simulink model "bh_compare_hand_to_SM_quad_pend"  (R2020b)
settings: Solver=ode23t  StartTime=0.0  StopTime=50  FixedStep=0.001  RelTol=1e-5  EnableMultiTasking=on
undefined symbols (not defined in the file): K, P_elec, P_mot, P_one_prop, P_pend, P_rot, P_veh, P_veh_no_props, sigbuilder_block, X, xme_dot_0, Y, Z
libraries: fl_lib x85, simulink_extras x42, nesl_utility x39, sm_lib x29, pid_lib x8, fl_ps_legacy_lib x7, simulink x6
(part 2 of 5)

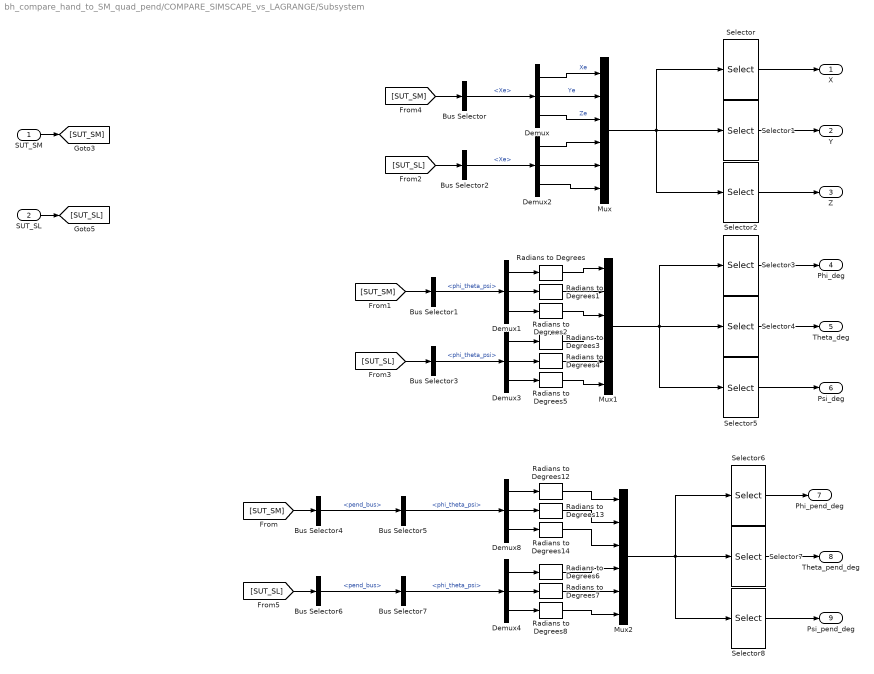
== system bh_compare_hand_to_SM_quad_pend/COMPARE_SIMSCAPE_vs_LAGRANGE/Subsystem ==
  SUT_SM : Inport
  SUT_SL : Inport  Port=2
  Bus Selector : BusSelector  OutputSignals=Xe
  Bus Selector{1,3,5,7} (4 alike) : BusSelector  OutputSignals=phi_theta_psi
  Bus Selector2 : BusSelector  OutputSignals=Xe
  Bus Selector4 : BusSelector  OutputSignals=pend_bus
  Bus Selector6 : BusSelector  OutputSignals=pend_bus
  Demux{,1..4,8} (6 alike) : Demux  Outputs=3
  Mux : Mux  Inputs=6
  Mux1 : Mux  Inputs=6
  Mux2 : Mux  Inputs=6
  Radians to Degrees{,1..8,12..14} (12 alike) : simulink_extras/Transformations/Radians to Degrees
  Selector : Selector  InputPortWidth=6  IndexOptions=Index vector (dialog)  Indices=[1 4]  OutputSizes=1
  Selector1 : Selector  InputPortWidth=6  IndexOptions=Index vector (dialog)  Indices=[2 5]  OutputSizes=1
  Selector2 : Selector  InputPortWidth=6  IndexOptions=Index vector (dialog)  Indices=[3 6]  OutputSizes=1
  Selector3 : Selector  InputPortWidth=6  IndexOptions=Index vector (dialog)  Indices=[1 4]  OutputSizes=1
  Selector4 : Selector  InputPortWidth=6  IndexOptions=Index vector (dialog)  Indices=[2 5]  OutputSizes=1
  Selector5 : Selector  InputPortWidth=6  IndexOptions=Index vector (dialog)  Indices=[3 6]  OutputSizes=1
  Selector6 : Selector  InputPortWidth=6  IndexOptions=Index vector (dialog)  Indices=[1 4]  OutputSizes=1
  Selector7 : Selector  InputPortWidth=6  IndexOptions=Index vector (dialog)  Indices=[2 5]  OutputSizes=1
  Selector8 : Selector  InputPortWidth=6  IndexOptions=Index vector (dialog)  Indices=[3 6]  OutputSizes=1
  X : Outport  VectorParamsAs1DForOutWhenUnconnected=off
  Y : Outport  Port=2  VectorParamsAs1DForOutWhenUnconnected=off
  Z : Outport  Port=3  VectorParamsAs1DForOutWhenUnconnected=off
  Phi_deg : Outport  Port=4  VectorParamsAs1DForOutWhenUnconnected=off
  Theta_deg : Outport  Port=5  VectorParamsAs1DForOutWhenUnconnected=off
  Psi_deg : Outport  Port=6  VectorParamsAs1DForOutWhenUnconnected=off
  Phi_pend_deg : Outport  Port=7  VectorParamsAs1DForOutWhenUnconnected=off
  Theta_pend_deg : Outport  Port=8  VectorParamsAs1DForOutWhenUnconnected=off
  Psi_pend_deg : Outport  Port=9  VectorParamsAs1DForOutWhenUnconnected=off
  wires:
  SUT_SL/1 -> [SUT_SL]
  SUT_SM/1 -> [SUT_SM]
  Demux8/2 -> Radians to Degrees13/1
  [SUT_SM] -> Bus Selector1/1
  Bus Selector1/1 -> Demux1/1  "<phi_theta_psi>"
  Bus Selector/1 -> Demux/1  "<Xe>"
  Demux1/2 -> Radians to Degrees1/1
  Demux8/3 -> Radians to Degrees14/1
  [SUT_SM] -> Bus Selector4/1
  Demux8/1 -> Radians to Degrees12/1
  [SUT_SM] -> Bus Selector/1
  Demux1/1 -> Radians to Degrees/1
  Demux1/3 -> Radians to Degrees2/1
  [SUT_SL] -> Bus Selector2/1
  Bus Selector2/1 -> Demux2/1  "<Xe>"
  Demux3/1 -> Radians to Degrees3/1
  [SUT_SL] -> Bus Selector3/1
  Bus Selector3/1 -> Demux3/1  "<phi_theta_psi>"
  Demux3/2 -> Radians to Degrees4/1
  Demux3/3 -> Radians to Degrees5/1
  Bus Selector4/1 -> Bus Selector5/1  "<pend_bus>"
  Bus Selector5/1 -> Demux8/1  "<phi_theta_psi>"
  [SUT_SL] -> Bus Selector6/1
  Demux4/2 -> Radians to Degrees7/1
  Demux4/1 -> Radians to Degrees6/1
  Demux4/3 -> Radians to Degrees8/1
  Bus Selector6/1 -> Bus Selector7/1  "<pend_bus>"
  Bus Selector7/1 -> Demux4/1  "<phi_theta_psi>"
  Demux2/2 -> Mux/5
  Demux2/3 -> Mux/6
  Demux2/1 -> Mux/4
  Demux/3 -> Mux/3  "Ze"
  Demux/2 -> Mux/2  "Ye"
  Demux/1 -> Mux/1  "Xe"
  Radians to Degrees5/1 -> Mux1/6
  Radians to Degrees4/1 -> Mux1/5
  Radians to Degrees3/1 -> Mux1/4
  Radians to Degrees2/1 -> Mux1/3
  Radians to Degrees1/1 -> Mux1/2
  Radians to Degrees/1 -> Mux1/1
  Radians to Degrees12/1 -> Mux2/1
  Radians to Degrees13/1 -> Mux2/2
  Radians to Degrees14/1 -> Mux2/3
  Radians to Degrees6/1 -> Mux2/4
  Radians to Degrees7/1 -> Mux2/5
  Radians to Degrees8/1 -> Mux2/6
  Mux2/1 -> Selector8/1, Selector6/1, Selector7/1
  Mux/1 -> Selector/1, Selector2/1, Selector1/1
  Mux1/1 -> Selector5/1, Selector3/1, Selector4/1
  Selector2/1 -> Z/1
  Selector1/1 -> Y/1
  Selector/1 -> X/1
  Selector5/1 -> Psi_deg/1
  Selector4/1 -> Theta_deg/1
  Selector3/1 -> Phi_deg/1
  Selector6/1 -> Phi_pend_deg/1
  Selector8/1 -> Psi_pend_deg/1
  Selector7/1 -> Theta_pend_deg/1

== system bh_compare_hand_to_SM_quad_pend/CONT_SYS W_MOT_CMDS1/MOTOR_sys ==
  w_CMD : Inport
  Demux : Demux
  MOTOR_1 : Subsystem
      mask Display: image('bh_PIC_MOTOR.jpg');
  MOTOR_2 : Subsystem
      mask Display: image('bh_PIC_MOTOR.jpg');
  MOTOR_3 : Subsystem
      mask Display: image('bh_PIC_MOTOR.jpg');
  MOTOR_4 : Subsystem
      mask Display: image('bh_PIC_MOTOR.jpg');
  Mux : Mux
  w CMD vs Actual : Scope  NumInputPorts=4
  w_MUX : Subsystem
  w : Outport  VectorParamsAs1DForOutWhenUnconnected=off
  wires:
  MOTOR_4/1(w) -> Mux/4
  MOTOR_3/1(w) -> Mux/3
  MOTOR_2/1(w) -> Mux/2
  MOTOR_1/1(w) -> Mux/1
  Demux/1 -> MOTOR_1/1(w_CMD)
  Demux/2 -> MOTOR_2/1(w_CMD)
  Demux/3 -> MOTOR_3/1(w_CMD)
  Demux/4 -> MOTOR_4/1(w_CMD)
  w_CMD/1 -> [W_CMD], Demux/1
  w_MUX/4(w4) -> w CMD vs Actual/4
  w_MUX/2(w2) -> w CMD vs Actual/2
  w_MUX/3(w3) -> w CMD vs Actual/3
  w_MUX/1(w1) -> w CMD vs Actual/1
  [W_CMD] -> w_MUX/1(W_CMD)
  Mux/1 -> w_MUX/2(W), w/1

== system bh_compare_hand_to_SM_quad_pend/CONT_SYS W_MOT_CMDS1/SIGN_CONVENTIONS ==

== system bh_compare_hand_to_SM_quad_pend/CONT_SYS W_MOT_CMDS1/W2_checker ==
  w2_CMD : Inport
  Assertion{,1..3} (4 alike) : Assertion
  Compare To Constant : simulink/Logic and Bit Operations/Compare To Constant  relop=>=  const=0  OutDataTypeStr=boolean
  Demux : Demux
  w2 : Outport  VectorParamsAs1DForOutWhenUnconnected=off
  wires:
  w2_CMD/1 -> w2/1, Compare To Constant/1
  Compare To Constant/1 -> Demux/1
  Demux/1 -> Assertion/1
  Demux/4 -> Assertion3/1
  Demux/3 -> Assertion2/1
  Demux/2 -> Assertion1/1

== system bh_compare_hand_to_SM_quad_pend/CONT_SYS W_MOT_CMDS1/w_to_RPS1 ==
  w : Inport
  Constant : Constant  Value=3.141592653589793
  Gain1 : Gain  Gain=2
  Product : Product  Inputs=*/
  RPS : Outport
  wires:
  Product/1 -> RPS/1
  Gain1/1 -> Product/2  "2PI"
  Constant/1 -> Gain1/1
  w/1 -> Product/1  "w_per_sec"

== system bh_compare_hand_to_SM_quad_pend/CONT_SYS W_MOT_CMDS2/PRE_FILTERS ==
  w_in : Inport
  Demux : Demux
  Mux : Mux
  Reshape2 : Reshape  OutputDimensionality=Column vector (2-D)
  Terminator{,1..3} (4 alike) : Terminator
  prefilter : Subsystem  mask(Derivative Estimation){wn=2*pi*5, p=1}
      mask prompts: wn "Natural frequency, wn (rad/sec)"; p "Damping ratio, p"
      mask help:
      | A simple derivative estimator using a 2nd order representation between input and output.
      |
      | The integrators use a discrete FORWARd Euler rule, and a sample time needs to be specified.
      mask init:
      | str1 = sprintf('wn = %.2f', wn);
      | str2 = sprintf('p  = %.2f', p);
      | %str3 = sprintf('dt = %.2f', dt);
      | %str = char(str1,str2,str3);
      | %str3 = sprintf('dt = %.2f', dt);
      | str = char(str1,str2);
      mask Display: disp(str)
  prefilter1 : Subsystem  mask(Derivative Estimation){wn=2*pi*5, p=1}
      mask prompts: wn "Natural frequency, wn (rad/sec)"; p "Damping ratio, p"
      mask help:
      | A simple derivative estimator using a 2nd order representation between input and output.
      |
      | The integrators use a discrete FORWARd Euler rule, and a sample time needs to be specified.
      mask init:
      | str1 = sprintf('wn = %.2f', wn);
      | str2 = sprintf('p  = %.2f', p);
      | %str3 = sprintf('dt = %.2f', dt);
      | %str = char(str1,str2,str3);
      | %str3 = sprintf('dt = %.2f', dt);
      | str = char(str1,str2);
      mask Display: disp(str)
  prefilter2 : Subsystem  mask(Derivative Estimation){wn=2*pi*5, p=1}
      mask prompts: wn "Natural frequency, wn (rad/sec)"; p "Damping ratio, p"
      mask help:
      | A simple derivative estimator using a 2nd order representation between input and output.
      |
      | The integrators use a discrete FORWARd Euler rule, and a sample time needs to be specified.
      mask init:
      | str1 = sprintf('wn = %.2f', wn);
      | str2 = sprintf('p  = %.2f', p);
      | %str3 = sprintf('dt = %.2f', dt);
      | %str = char(str1,str2,str3);
      | %str3 = sprintf('dt = %.2f', dt);
      | str = char(str1,str2);
      mask Display: disp(str)
  prefilter3 : Subsystem  mask(Derivative Estimation){wn=2*pi*5, p=1}
      mask prompts: wn "Natural frequency, wn (rad/sec)"; p "Damping ratio, p"
      mask help:
      | A simple derivative estimator using a 2nd order representation between input and output.
      |
      | The integrators use a discrete FORWARd Euler rule, and a sample time needs to be specified.
      mask init:
      | str1 = sprintf('wn = %.2f', wn);
      | str2 = sprintf('p  = %.2f', p);
      | %str3 = sprintf('dt = %.2f', dt);
      | %str = char(str1,str2,str3);
      | %str3 = sprintf('dt = %.2f', dt);
      | str = char(str1,str2);
      mask Display: disp(str)
  w CMD vs Actual : Scope  NumInputPorts=4
  w_MUX : Subsystem
  w : Outport  VectorParamsAs1DForOutWhenUnconnected=off
  wires:
  prefilter1/2(U_DOT) -> Terminator1/1
  prefilter/2(U_DOT) -> Terminator/1
  prefilter2/2(U_DOT) -> Terminator2/1
  prefilter3/2(U_DOT) -> Terminator3/1
  w_in/1 -> [W_CMD], Demux/1
  Demux/1 -> prefilter/1(U)
  Demux/2 -> prefilter1/1(U)
  Demux/3 -> prefilter2/1(U)
  Demux/4 -> prefilter3/1(U)
  prefilter/1(U_filt) -> Mux/1
  prefilter1/1(U_filt) -> Mux/2
  prefilter2/1(U_filt) -> Mux/3
  prefilter3/1(U_filt) -> Mux/4
  Mux/1 -> Reshape2/1
  Reshape2/1 -> w_MUX/2(W), w/1
  w_MUX/3(w3) -> w CMD vs Actual/3
  w_MUX/2(w2) -> w CMD vs Actual/2
  w_MUX/4(w4) -> w CMD vs Actual/4
  [W_CMD] -> w_MUX/1(W_CMD)
  w_MUX/1(w1) -> w CMD vs Actual/1

== system bh_compare_hand_to_SM_quad_pend/CONT_SYS W_MOT_CMDS2/SIGN_CONVENTIONS ==

== system bh_compare_hand_to_SM_quad_pend/CONT_SYS W_MOT_CMDS2/W2_checker ==
  w2_CMD : Inport
  Assertion{,1..3} (4 alike) : Assertion
  Compare To Constant : simulink/Logic and Bit Operations/Compare To Constant  relop=>=  const=0  OutDataTypeStr=boolean
  Demux : Demux
  w2 : Outport  VectorParamsAs1DForOutWhenUnconnected=off
  wires:
  w2_CMD/1 -> w2/1, Compare To Constant/1
  Compare To Constant/1 -> Demux/1
  Demux/1 -> Assertion/1
  Demux/4 -> Assertion3/1
  Demux/3 -> Assertion2/1
  Demux/2 -> Assertion1/1

== system bh_compare_hand_to_SM_quad_pend/CONT_SYS W_MOT_CMDS2/w_to_RPS1 ==
  w : Inport
  Constant : Constant  Value=3.141592653589793
  Gain1 : Gain  Gain=2
  Product : Product  Inputs=*/
  RPS : Outport
  wires:
  Product/1 -> RPS/1
  Gain1/1 -> Product/2  "2PI"
  Constant/1 -> Gain1/1
  w/1 -> Product/1  "w_per_sec"

== system bh_compare_hand_to_SM_quad_pend/EYES_PROP_and_VEH/THRUST_FUSE ==
  REF : Inport
  p1_b : Inport  Port=2
  p2_b : Inport  Port=3
  p3_b : Inport  Port=4
  p4_b : Inport  Port=5
  Bus Selector{,1..3} (4 alike) : BusSelector  OutputSignals=Thrust_on_veh
  Mux{,1..3} (4 alike) : Mux  Inputs=2
  Selector : Selector  InputPortWidth=4  IndexOptions=Index vector (dialog)  Indices=1  OutputSizes=1
  Selector1 : Selector  InputPortWidth=4  IndexOptions=Index vector (dialog)  Indices=2  OutputSizes=1
  Selector2 : Selector  InputPortWidth=4  IndexOptions=Index vector (dialog)  Indices=3  OutputSizes=1
  Selector3 : Selector  InputPortWidth=4  IndexOptions=Index vector (dialog)  Indices=4  OutputSizes=1
  Out1 : Outport  VectorParamsAs1DForOutWhenUnconnected=off
  Out2 : Outport  Port=2  VectorParamsAs1DForOutWhenUnconnected=off
  Out3 : Outport  Port=3  VectorParamsAs1DForOutWhenUnconnected=off
  Out4 : Outport  Port=4  VectorParamsAs1DForOutWhenUnconnected=off
  wires:
  Mux/1 -> Out4/1
  Mux1/1 -> Out3/1
  Mux2/1 -> Out2/1
  Mux3/1 -> Out1/1
  p1_b/1 -> Bus Selector/1
  Bus Selector/1 -> Mux3/2  "<Thrust_on_veh>"
  Selector/1 -> Mux3/1
  Selector1/1 -> Mux2/1
  Selector2/1 -> Mux1/1
  Selector3/1 -> Mux/1
  REF/1 -> Selector3/1, Selector2/1, Selector1/1, Selector/1
  p2_b/1 -> Bus Selector1/1
  Bus Selector1/1 -> Mux2/2  "<Thrust_on_veh>"
  p3_b/1 -> Bus Selector2/1
  Bus Selector2/1 -> Mux1/2  "<Thrust_on_veh>"
  p4_b/1 -> Bus Selector3/1
  Bus Selector3/1 -> Mux/2  "<Thrust_on_veh>"

== system bh_compare_hand_to_SM_quad_pend/EYES_PROP_and_VEH/TQ_FUSE ==
  REF : Inport
  p1_b : Inport  Port=2
  p2_b : Inport  Port=3
  p3_b : Inport  Port=4
  p4_b : Inport  Port=5
  Bus Selector{,1..3} (4 alike) : BusSelector  OutputSignals=Torque_on_veh
  Mux{,1..3} (4 alike) : Mux  Inputs=2
  Selector : Selector  InputPortWidth=4  IndexOptions=Index vector (dialog)  Indices=1  OutputSizes=1
  Selector1 : Selector  InputPortWidth=4  IndexOptions=Index vector (dialog)  Indices=2  OutputSizes=1
  Selector2 : Selector  InputPortWidth=4  IndexOptions=Index vector (dialog)  Indices=3  OutputSizes=1
  Selector3 : Selector  InputPortWidth=4  IndexOptions=Index vector (dialog)  Indices=4  OutputSizes=1
  Out1 : Outport  VectorParamsAs1DForOutWhenUnconnected=off
  Out2 : Outport  Port=2  VectorParamsAs1DForOutWhenUnconnected=off
  Out3 : Outport  Port=3  VectorParamsAs1DForOutWhenUnconnected=off
  Out4 : Outport  Port=4  VectorParamsAs1DForOutWhenUnconnected=off
  wires:
  Mux/1 -> Out4/1
  Mux1/1 -> Out3/1
  Mux2/1 -> Out2/1
  Mux3/1 -> Out1/1
  p1_b/1 -> Bus Selector/1
  Bus Selector/1 -> Mux3/2  "<Torque_on_veh>"
  Selector/1 -> Mux3/1
  Selector1/1 -> Mux2/1
  Selector2/1 -> Mux1/1
  Selector3/1 -> Mux/1
  REF/1 -> Selector3/1, Selector2/1, Selector1/1, Selector/1
  p2_b/1 -> Bus Selector1/1
  Bus Selector1/1 -> Mux2/2  "<Torque_on_veh>"
  p3_b/1 -> Bus Selector2/1
  Bus Selector2/1 -> Mux1/2  "<Torque_on_veh>"
  p4_b/1 -> Bus Selector3/1
  Bus Selector3/1 -> Mux/2  "<Torque_on_veh>"

== system bh_compare_hand_to_SM_quad_pend/EYES_PROP_and_VEH/w_FUSE ==
  REF : Inport
  p1_b : Inport  Port=2
  p2_b : Inport  Port=3
  p3_b : Inport  Port=4
  p4_b : Inport  Port=5
  Bus Selector{,1..3} (4 alike) : BusSelector  OutputSignals=w_prop
  Mux{,1..3} (4 alike) : Mux  Inputs=2
  Selector : Selector  InputPortWidth=4  IndexOptions=Index vector (dialog)  Indices=1  OutputSizes=1
  Selector1 : Selector  InputPortWidth=4  IndexOptions=Index vector (dialog)  Indices=2  OutputSizes=1
  Selector2 : Selector  InputPortWidth=4  IndexOptions=Index vector (dialog)  Indices=3  OutputSizes=1
  Selector3 : Selector  InputPortWidth=4  IndexOptions=Index vector (dialog)  Indices=4  OutputSizes=1
  Out1 : Outport  VectorParamsAs1DForOutWhenUnconnected=off
  Out2 : Outport  Port=2  VectorParamsAs1DForOutWhenUnconnected=off
  Out3 : Outport  Port=3  VectorParamsAs1DForOutWhenUnconnected=off
  Out4 : Outport  Port=4  VectorParamsAs1DForOutWhenUnconnected=off
  wires:
  Mux/1 -> Out4/1
  Mux1/1 -> Out3/1
  Mux2/1 -> Out2/1
  Mux3/1 -> Out1/1
  p1_b/1 -> Bus Selector/1
  Bus Selector/1 -> Mux3/2  "<w_prop>"
  Selector/1 -> Mux3/1
  Selector1/1 -> Mux2/1
  Selector2/1 -> Mux1/1
  Selector3/1 -> Mux/1
  REF/1 -> Selector3/1, Selector2/1, Selector1/1, Selector/1
  Bus Selector1/1 -> Mux2/2  "<w_prop>"
  p2_b/1 -> Bus Selector1/1
  Bus Selector2/1 -> Mux1/2  "<w_prop>"
  p3_b/1 -> Bus Selector2/1
  Bus Selector3/1 -> Mux/2  "<w_prop>"
  p4_b/1 -> Bus Selector3/1

== system bh_compare_hand_to_SM_quad_pend/MODEL_SYS/SIGN_CONVENTIONS ==

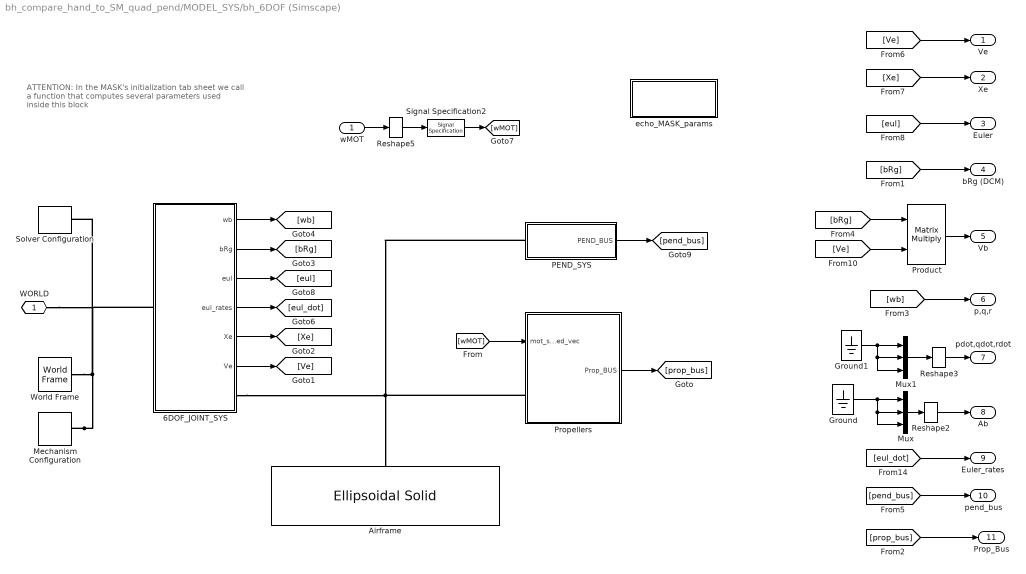
== system bh_compare_hand_to_SM_quad_pend/MODEL_SYS/bh_6DOF (Simscape) ==
  note: ATTENTION:
      | In the MASK's initialization tab sheet
      | we call a function that computes several parameters
      | used inside this block
  wMOT : Inport
  6DOF_JOINT_SYS : Subsystem
  Airframe : sm_lib/Body Elements/Ellipsoidal Solid  GraphicAmbientColor=[0.15 0.15 0.15 1.0]  BasedOnType=Density  CenterOfMass=[0 0 0]  CenterOfMassUnits=m  GraphicDiffuseColor=[0.5 0.5 0.5]  Density=1000  DensityUnits=kg/(m^3)  DoExposeReferenceFrame=on  EllipsoidRadii=[prop_CG_L, prop_CG_L, prop_CG_L/10]  EllipsoidRadiiUnits=m  GraphicEmissiveColor=[0.0 0.0 0.0 1.0]  ExportEntireGeometry=off  SerializedFrames=<Frames/>  MarkerShape=Sphere  MarkerSize=10  GraphicType=FromGeometry  InertiaType=Custom  Mass=air_mass_0  MassUnits=kg  MomentsOfInertia=Iair_xx_yy_zz  MomentsOfInertiaUnits=kg*m^2  GraphicOpacity=1.0  ProductsOfInertia=Iair_yz_zx_xy  ProductsOfInertiaUnits=kg*m^2  GraphicShininess=75  GraphicSpecularColor=[0.5 0.5 0.5 1.0]  GraphicVisPropType=SimpleVisualProperties
      settings: SourceProductBaseCode=MS
      settings: AttributesFormatString=|
      | %<Mass>
      | %<MomentsOfInertia>
      | %<ProductsOfInertia>
  Ground : Ground
  Ground1 : Ground
  Mechanism Configuration : sm_lib/Utilities/Mechanism Configuration  UniformGravity=Constant  GravityVector=[0, 0, -g_const]  GravityVectorUnits=m/s^2  GravityUnits=m/s^2  LinearizationDelta=0.001  JointModeTransitionNonlinearIterations=2
  Mux : Mux  Inputs=3
  Mux1 : Mux  Inputs=3
  PEND_SYS : Subsystem
  Product : Product  Multiplication=Matrix(*)
  Propellers : Subsystem
  Reshape2 : Reshape  OutputDimensionality=Column vector (2-D)
  Reshape3 : Reshape  OutputDimensionality=Column vector (2-D)
  Reshape5 : Reshape  OutputDimensionality=Column vector (2-D)
  Signal Specification2 : SignalSpecification  Dimensions=[4,1]
  Solver Configuration : nesl_utility/Solver Configuration  PhysicalDomain=network_engine_domain  SubClassName=solver  LeftPortType=input  RightPortType=generic  Tones=[]  Harmonics=[]  SimulateNoise=off  Profile=off  UseLocalSampling=off  EnableSwitchedLinearOptims=on  FrequencyDomain=off  UseCCode=off  RelTol=0.001  AbsTol=1e-06  MinStep=1e-09  ToWorkspace=off  RevertToSquareIcSolve=off  NumHomotopyIterations=100  PhasorMode=off  PhasorModeNumHarmonics=1  DoDC=off  ResidualTolerance=1e-09  UseLocalSolver=off  LocalSolverChoice=NE_BACKWARD_EULER_ADVANCER  LocalSolverSampleTime=0.001  DoFixedCost=off  MaxNonlinIter=3  MaxModeIter=2  ComputeImpulses=off  ImpulseIterations=2  LinearAlgebra=Sparse  EquationFormulation=NE_TIME_EF  DelaysMemoryBudget=1024  AutomaticFiltering=on  FilteringTimeConstant=0.001  PartitionStorageMethod=AS_NEEDED  PartitionMemoryBudget=1024  PartitionMethod=FAST
  World Frame : sm_lib/Frames and Transforms/World Frame
  echo_MASK_params : Subsystem
  WORLD : PMIOPort  Side=Left
  Ve : Outport  VectorParamsAs1DForOutWhenUnconnected=off
  Xe : Outport  Port=2  VectorParamsAs1DForOutWhenUnconnected=off
  Euler : Outport  Port=3  VectorParamsAs1DForOutWhenUnconnected=off
  bRg (DCM) : Outport  Port=4  VectorParamsAs1DForOutWhenUnconnected=off
  Vb : Outport  Port=5  VectorParamsAs1DForOutWhenUnconnected=off
  p,q,r : Outport  Port=6  VectorParamsAs1DForOutWhenUnconnected=off
  pdot,qdot,rdot : Outport  Port=7  VectorParamsAs1DForOutWhenUnconnected=off
  Ab : Outport  Port=8  VectorParamsAs1DForOutWhenUnconnected=off
  Euler_rates : Outport  Port=9  VectorParamsAs1DForOutWhenUnconnected=off
  pend_bus : Outport  Port=10  VectorParamsAs1DForOutWhenUnconnected=off
  Prop_Bus : Outport  Port=11  VectorParamsAs1DForOutWhenUnconnected=off
  wires:
  [Ve] -> Ve/1
  [Xe] -> Xe/1
  [eul] -> Euler/1
  [bRg] -> bRg (DCM)/1
  Mux/1 -> Reshape2/1
  Reshape2/1 -> Ab/1
  Ground/1 -> Mux/2, Mux/3, Mux/1
  Product/1 -> Vb/1
  [wb] -> p,q,r/1
  [eul_dot] -> Euler_rates/1
  Ground1/1 -> Mux1/2, Mux1/3, Mux1/1
  Reshape3/1 -> pdot,qdot,rdot/1
  Mux1/1 -> Reshape3/1
  wMOT/1 -> Reshape5/1
  Reshape5/1 -> Signal Specification2/1
  Signal Specification2/1 -> [wMOT]
  [wMOT] -> Propellers/1(mot_speed_vec)
  6DOF_JOINT_SYS/2(bRg) -> [bRg]
  6DOF_JOINT_SYS/5(Xe) -> [Xe]
  6DOF_JOINT_SYS/6(Ve) -> [Ve]
  6DOF_JOINT_SYS/1(wb) -> [wb]
  [Ve] -> Product/2
  [bRg] -> Product/1
  6DOF_JOINT_SYS/4(eul_rates) -> [eul_dot]
  6DOF_JOINT_SYS/3(eul) -> [eul]
  PEND_SYS/1(PEND_BUS) -> [pend_bus]
  [pend_bus] -> pend_bus/1
  Propellers/1(Prop_BUS) -> [prop_bus]
  [prop_bus] -> Prop_Bus/1
  connections:
  Mechanism Configuration/RConn1 -- WORLD/RConn1 -- 6DOF_JOINT_SYS/LConn1 -- Solver Configuration/RConn1 -- World Frame/RConn1
  6DOF_JOINT_SYS/RConn1 -- Airframe/RConn1 -- Propellers/LConn1 -- PEND_SYS/LConn1

== system bh_compare_hand_to_SM_quad_pend/SAR/XYZ_CMDS ==
  Demux : Demux  Tag=STV Demux  Outputs=3
      settings: DisplayOption=none
  FromWs : FromWorkspace  Tag=STV FromWs  VariableName=tuvar
      SigBuilderData=|
      | common.afterFinalStr = 'Extrapolate'
      | common.sampleTime = 0
      | dataSet(1).timeRange = [0 200]
      | dataSet(1).name = 'small_steps'
      | dataSet(2).timeRange = [0 200]
      | dataSet(2).name = 'zStairs_xyConstVEL'
      | dataSet(3).timeRange = [0 500]
      | dataSet(3).name = 'sineWaves'
      | dataSet(4).timeRange = [0 200]
      | dataSet(4).name = 'ZERO'
      | dataSet(5).timeRange = [0 200]
      | dataSet(5).name = 'SEARCH_P1'
      | sbobj.Name = 'Signal Builder'
      | sbobj.Groups(1).Name = 'small_steps'
      | sbobj.Groups(1).Signals(1).Name = 'Z'
      | sbobj.Groups(1).Signals(1).XData = [0 10 10.000001 20 20.000001 30 30.000001 55 200]
      | sbobj.Groups(1).Signals(1).YData = [0 0 2 2 2 2 2 2 2]
      | sbobj.Groups(1).Signals(2).Name = 'X'
      | sbobj.Groups(1).Signals(2).XData = [0 10 10.000001 20 20.000001 30 30.000001 55 200]
      | sbobj.Groups(1).Signals(2).YData = [0 0 0 0 3 3 3 3 3]
      | sbobj.Groups(1).Signals(3).Name = 'Y'
      | sbobj.Groups(1).Signals(3).XData = [0 10 10.000001 20 20.000001 30 30.000001 55 200]
      | sbobj.Groups(1).Signals(3).YData = [0 0 0 0 0 0 1 1 1]
      | sbobj.Groups(1).TimeRange = [0 200]
      | sbobj.Groups(2).Name = 'zStairs_xyConstVEL'
      | sbobj.Groups(2).Signals(1).Name = 'Z'
      | sbobj.Groups(2).Signals(1).XData = [0 10 10.000001 20 20.000001 30 30.000001 40 40.000001 55 200]
      | sbobj.Groups(2).Signals(1).YData = [0 0 1 1 2 2 1 1 0 0 0]
      | sbobj.Groups(2).Signals(2).Name = 'X'
      | sbobj.Groups(2).Signals(2).XData = [0 10 10.000001 20 20.000001 30 30.000001 40 40.000001 55 200]
      | sbobj.Groups(2).Signals(2).YData = [0 1 1.0000001 2 2.0000001 3 3.0000001 4 4.0000001 5.5 20]
      | sbobj.Groups(2).Signals(3).Name = 'Y'
      | sbobj.Groups(2).Signals(3).XData = [0 10 10.000001 20 20.000001 30 30.000001 40 40.000001 55 200]
      | sbobj.Groups(2).Signals(3).YData = [0 0.5 0.50000005 1 1.00000005 1.5 1.50000005 2 2.00000005 2.75 10]
      | sbobj.Groups(2).TimeRange = [0 200]
      | sbobj.Groups(3).Name = 'sineWaves'
      | sbobj.Groups(3).Signals(1).Name = 'Z'
      | sbobj.Groups(3).Signals(1).XData = [0 0.1 0.2 0.3 0.4 0.5 0.6 0.7 0.8 0.9 1 1.1 ... (5001 elements, 1x5001)]
      | sbobj.Groups(3).Signals(1).YData = [0 0.0314107325553 0.0627904665622 0.0941082340641 0.125333128258 0.156434333994 0.18738115819 0.218143060119 0.248689681547 0.278990876699 0.309016742004 0.338737645607 ... (5001 elements, 1x5001)]
      | sbobj.Groups(3).Signals(2).Name = 'X'
      | sbobj.Groups(3).Signals(2).XData = [0 0.1 0.2 0.3 0.4 0.5 0.6 0.7 0.8 0.9 1 1.1 ... (5001 elements, 1x5001)]
      | sbobj.Groups(3).Signals(2).YData = [0 0.01 0.02 0.03 0.04 0.05 0.06 0.07 0.08 0.09 0.1 0.11 ... (5001 elements, 1x5001)]
      | sbobj.Groups(3).Signals(3).Name = 'Y'
      | sbobj.Groups(3).Signals(3).XData = [0 0.1 0.2 0.3 0.4 0.5 0.6 0.7 0.8 0.9 1 1.1 ... (5001 elements, 1x5001)]
      | sbobj.Groups(3).Signals(3).YData = [0 0.0157073040455 0.0314107325553 0.04710641095 0.0627904665622 0.0784590295926 0.0941082340641 0.109734218776 0.125333128258 0.140901113717 0.156434333994 0.171928956505 ... (5001 elements, 1x5001)]
      | sbobj.Groups(3).TimeRange = [0 500]
      | sbobj.Groups(4).Name = 'ZERO'
      | sbobj.Groups(4).Signals(1).Name = 'Z'
      | sbobj.Groups(4).Signals(1).XData = [0 200]
      | sbobj.Groups(4).Signals(1).YData = [0 0]
      | sbobj.Groups(4).Signals(2).Name = 'X'
      | sbobj.Groups(4).Signals(2).XData = [0 200]
      | sbobj.Groups(4).Signals(2).YData = [0 0]
      | sbobj.Groups(4).Signals(3).Name = 'Y'
      | sbobj.Groups(4).Signals(3).XData = [0 200]
      | sbobj.Groups(4).Signals(3).YData = [0 0]
      | sbobj.Groups(4).TimeRange = [0 200]
      | sbobj.Groups(5).Name = 'SEARCH_P1'
      | sbobj.Groups(5).Signals(1).Name = 'Z'
      | sbobj.Groups(5).Signals(1).XData = [0 7 27 32 52 57 77 82 102 107 127 132 157 187 200]
      | sbobj.Groups(5).Signals(1).YData = [0 5 5 5 5 5 5 5 5 5 5 5 5 0 0]
      | sbobj.Groups(5).Signals(2).Name = 'X'
      | sbobj.Groups(5).Signals(2).XData = [0 7 27 32 52 57 77 82 102 107 127 132 157 187 200]
      | sbobj.Groups(5).Signals(2).YData = [0 5 25 25 5 5 25 25 5 5 25 25 0 0 0]
      | sbobj.Groups(5).Signals(3).Name = 'Y'
      | sbobj.Groups(5).Signals(3).XData = [0 7 27 32 52 57 77 82 102 107 127 132 157 187 200]
      | sbobj.Groups(5).Signals(3).YData = [0 5 5 10 10 15 15 20 20 25 25 30 30 0 0]
      | sbobj.Groups(5).TimeRange = [0 200]
  Z : Outport  VectorParamsAs1DForOutWhenUnconnected=off
  X : Outport  Tag=STV Outport  Port=2  VectorParamsAs1DForOutWhenUnconnected=off
  Y : Outport  Tag=STV Outport  Port=3  VectorParamsAs1DForOutWhenUnconnected=off
  wires:
  Demux/1 -> Z/1
  FromWs/1 -> Demux/1
  Demux/2 -> X/1
  Demux/3 -> Y/1

== system bh_compare_hand_to_SM_quad_pend/XYZ CMD_LIMITS/prefilter ==
  note: Y = U *     wn^2/( s^2 + 2*p*wn*s + wn^2)
      | Y*( s^2 + 2*p*wn*s + wn^2) = U * wn^2
      |
      | y'' + y'*2*p*wn + y*wn^2 = U*wn^2
  U : Inport
  Gain : Gain  Gain=2*p*wn
  Gain1 : Gain  Gain=wn^2
  Gain2 : Gain  Gain=wn^2
  Integrator : Integrator
  Integrator1 : Integrator
  Sum : Sum  Inputs=|+--
  U_filt : Outport  VectorParamsAs1DForOutWhenUnconnected=off
  U_DOT : Outport  Port=2  VectorParamsAs1DForOutWhenUnconnected=off
  wires:
  Integrator/1 -> Integrator1/1, [Y_DOT], Gain/1  "y_dot"
  Sum/1 -> Integrator/1  "y_dot_dot"
  Integrator1/1 -> Gain1/1, U_filt/1  "y"
  U/1 -> Gain2/1
  Gain2/1 -> Sum/1
  Gain/1 -> Sum/3
  Gain1/1 -> Sum/2
  [Y_DOT] -> U_DOT/1

== system bh_compare_hand_to_SM_quad_pend/a_circle1/Signal Builder ==
  Demux : Demux  Tag=STV Demux  Outputs=2
      settings: DisplayOption=none
  FromWs : FromWorkspace  Tag=STV FromWs  VariableName=tuvar
      SigBuilderData=|
      | common.afterFinalStr = 'Extrapolate'
      | common.sampleTime = 0
      | dataSet.timeRange = [0 22]
      | dataSet.name = 'Group 1'
      | sbobj.Groups.Name = 'Group 1'
      | sbobj.Groups.Signals(1).Name = 'Signal 1'
      | sbobj.Groups.Signals(1).XData = [0 7.95 7.95 22]
      | sbobj.Groups.Signals(1).YData = [0 0 1.99 1.98]
      | sbobj.Groups.Signals(2).Name = 'Signal 2'
      | sbobj.Groups.Signals(2).XData = [0 12 16 22]
      | sbobj.Groups.Signals(2).YData = [0 0 1 1]
      | sbobj.Groups.TimeRange = [0 22]
  Signal 1 : Outport  Tag=STV Outport  VectorParamsAs1DForOutWhenUnconnected=off
  Signal 2 : Outport  Tag=STV Outport  Port=2  VectorParamsAs1DForOutWhenUnconnected=off
  wires:
  Demux/1 -> Signal 1/1
  FromWs/1 -> Demux/1
  Demux/2 -> Signal 2/1

== system bh_compare_hand_to_SM_quad_pend/a_circle1/Subsystem ==
  RPS : Inport
  Constant : Constant  Value=2*pi
  Product : Product  Inputs=**
  w_rad_psec : Outport  VectorParamsAs1DForOutWhenUnconnected=off
  wires:
  Constant/1 -> Product/2
  RPS/1 -> Product/1
  Product/1 -> w_rad_psec/1

== system bh_compare_hand_to_SM_quad_pend/CONT_SYS W_MOT_CMDS1/MOTOR_sys/MOTOR_1 ==
  note: motor with PROPELLER
  w_CMD : Inport
  Bus Selector1 : BusSelector  OutputSignals=Elec.i,TQ_mot.Kt_i
  Lift : Scope  NumInputPorts=3
  MOTOR_PARAMS_STRUCT : Subsystem  mask(DC motor){K=P_mot.Ka, B=P_mot.b, J=P_mot.I, GearRatio=1, R=P_mot.R, L=P_mot.L, Kb=P_mot.Ke, ID=P_mot.ID}
      mask prompts: K "Torque constant (N.m/A)"; B "Viscous friction co-efficient (N.m.s)"; J "Rotor Inertia (kg.m^2)"; GearRatio "Gear ratio (w_motor/w_wheel)"; R "Armature resistance (ohms)"; L "Armature Inductance (Henry)"; Kb "Back Emf constant (V.sec/rad)"; ID "Motor_ID  (#1 to #4)"
      mask help: DC motor
      mask DialogControl Container4 Prompt: Mechanical
      mask DialogControl Container9 Prompt: Electrical
      mask DialogControl Container32 Prompt: ID
      mask Display: disp('DC motor')
  Mux : Mux  Inputs=2
  PI_CONT : pid_lib/PID Controller  Controller=PI  Form=Parallel  TimeDomain=Continuous-time  UseExternalTs=off  SampleTime=-1  IntegratorMethod=Forward Euler  FilterMethod=Forward Euler  ControllerParametersSource=internal  P=2.97678216835849  I=24.9655384194189  D=-0.0417302954853434  UseFilter=on  N=6.67624174583517  TunerSelectOption=Transfer Function Based (PID Tuner App)  InitialConditionSource=internal  InitialConditionForIntegrator=0  InitialConditionForFilter=0  DifferentiatorICPrevScaledInput=0  ExternalReset=none  TrackingMode=off  Kt=1  LimitOutput=off  SatLimitsSource=internal  UpperSaturationLimit=inf  LowerSaturationLimit=-inf  LinearizeAsGain=on  AntiWindupMode=none  Kb=1  POutMin=[]  POutMax=[]  IOutMin=[]  IOutMax=[]  DOutMin=[]  DOutMax=[]  NOutMin=[]  NOutMax=[]  SumOutMin=[]  SumOutMax=[]  SaturationOutMin=[]  SaturationOutMax=[]  PParamMin=[]  PParamMax=[]  IParamMin=[]  IParamMax=[]  DParamMin=[]  DParamMax=[]  NParamMin=[]  NParamMax=[]  KbParamMin=[]  KbParamMax=[]  KtParamMin=[]  KtParamMax=[]  KbOutMin=[]  KbOutMax=[]  KtOutMin=[]  KtOutMax=[]  IntegratorOutMin=[]  IntegratorOutMax=[]  FilterOutMin=[]  FilterOutMax=[]  SumI1OutMin=[]  SumI1OutMax=[]  SumI2OutMin=[]  SumI2OutMax=[]  SumI3OutMin=[]  SumI3OutMax=[]  SumI4OutMin=[]  SumI4OutMax=[]  SumDOutMin=[]  SumDOutMax=[]  DifferentiatorOutMin=[]  DifferentiatorOutMax=[]  FilterDiffOutCoefMin=[]  FilterDiffOutCoefMax=[]  ReciprocalOutMin=[]  ReciprocalOutMax=[]  SumDenOutMin=[]  SumDenOutMax=[]  SumNumOutMin=[]  SumNumOutMax=[]  DivideOutMin=[]  DivideOutMax=[]  UdiffTsProdOutMin=[]  UdiffTsProdOutMax=[]  NTsProdOutMin=[]  NTsProdOutMax=[]  UintegralTsProdOutMin=[]  UintegralTsProdOutMax=[]  UngainTsProdOutMin=[]  UngainTsProdOutMax=[]  IntegratorContinuousStateAttributes=''  IntegratorStateMustResolveToSignalObject=off  IntegratorRTWStateStorageClass=Auto  FilterContinuousStateAttributes=''  FilterStateMustResolveToSignalObject=off  FilterRTWStateStorageClass=Auto  ParallelPVariant=InternalParameters  IdealPVariant=Disabled  IVariant=InternalParameters  DVariant=Disabled  IntegratorVariant=Continuous  SatVariant=Disabled  AWVariant=Passthrough  PCopyVariant=Disabled  TRVariant=Disabled  FdbkBlocksVariant=Forward  IdealPFdbkVariant=Disabled  SatFdbkVariant=Disabled  DerivativeFilterVariant=Disabled  NVariant=Disabled  NCopyVariant=Disabled_SignalSpec  FilterICVariant=Disabled  IntegratorICVariant=InternalICs  ExternalResetVariant=Disabled  TRSumVariant=Passthrough  SumFdbkVariant=Disabled  SumVariant=Sum_PI  TsampFilterVariant=InternalTs  TsampNgainVariant=Passthrough  TsampIntegralVariant=Passthrough  ExternalSaturationOutDataTypeStr=Inherit: Same as second input
  RPS_Lift_TG_drag : Scope  NumInputPorts=3
  Scope3 : Scope  NumInputPorts=4
  Sum1 : Sum  Inputs=|+-
  Terminator : Terminator
  VOLTAGE Saturation : Saturate  UpperLimit=P_elec.V_mot_max  LowerLimit=P_elec.V_mot_min
      settings: AttributesFormatString=|
      | Vmax = %<UpperLimit>
      | Vmin = %<LowerLimit>
  prefilter : Subsystem  mask(Derivative Estimation){wn=2*pi*5, p=1}
      mask prompts: wn "Natural frequency, wn (rad/sec)"; p "Damping ratio, p"
      mask help:
      | A simple derivative estimator using a 2nd order representation between input and output.
      |
      | The integrators use a discrete FORWARd Euler rule, and a sample time needs to be specified.
      mask init:
      | str1 = sprintf('wn = %.2f', wn);
      | str2 = sprintf('p  = %.2f', p);
      | %str3 = sprintf('dt = %.2f', dt);
      | %str = char(str1,str2,str3);
      | %str3 = sprintf('dt = %.2f', dt);
      | str = char(str1,str2);
      mask Display: disp(str)
  w_to_RPS : Subsystem
      mask Display: fprintf('w(rad/sec)\nto\nRPS')
  w_to_RPS1 : Subsystem
      mask Display: fprintf('w(rad/sec)\nto\nRPS')
  w_to_TQ_drag : Subsystem  mask(w_to_TQdrag){k=P_one_prop.TWIST_per_w2}
      mask prompts: k "k (N/ ( rad/sec)^2 )"
      mask help:
      | Convert angular speed w(rad/sec) into drag TORQUE,  M (N.m).
      | A simple quadratic rule is used:
      |
      | M = k * w^2
  w_to_Thrust : Subsystem  mask(w_to_thrust){k=P_one_prop.LIFT_per_w2}
      mask prompts: k "k (N/ ( rad/sec)^2 )"
      mask help:
      | Convert angular speed w(rad/sec) into lift thrust F (N).
      | A simple quadratic rule is used:
      |
      | F = k * w^2
  w : Outport  VectorParamsAs1DForOutWhenUnconnected=off
  wires:
  VOLTAGE Saturation/1 -> Lift/1, MOTOR_PARAMS_STRUCT/1(V)  "VOLTS"
  [TQdrag] -> RPS_Lift_TG_drag/3  "TQdrag"
  Sum1/1 -> PI_CONT/1
  w_to_TQ_drag/1(M) -> [TQdrag], MOTOR_PARAMS_STRUCT/2(TQ_LOAD), Scope3/4
  [LIFT] -> RPS_Lift_TG_drag/2  "LIFT"
  [wRPS_YES_prop] -> RPS_Lift_TG_drag/1  "RPS"
  w_to_Thrust/1(F) -> [LIFT]
  w_to_RPS/1(RPS) -> [wRPS_YES_prop], Scope3/1  "RPS"
  Bus Selector1/1 -> Scope3/2  "<i>"
  MOTOR_PARAMS_STRUCT/2(mot_bus) -> Bus Selector1/1
  Bus Selector1/2 -> Scope3/3  "<Kt_i>"
  MOTOR_PARAMS_STRUCT/1(w_motor) -> w_to_RPS/1(w), [w], w/1, w_to_Thrust/1(w), w_to_TQ_drag/1(w)
  [w] -> Sum1/2
  [LIFT] -> Lift/2  "LIFT"
  Mux/1 -> w_to_RPS1/1(w)  "w"
  [w] -> Mux/2
  w_to_RPS1/1(RPS) -> Lift/3  "w_RPS"
  PI_CONT/1 -> VOLTAGE Saturation/1  "VOLTS"
  w_CMD/1 -> prefilter/1(U)  "w_rad_per_sec"
  prefilter/1(U_filt) -> Mux/1, Sum1/1
  prefilter/2(U_DOT) -> Terminator/1

== system bh_compare_hand_to_SM_quad_pend/CONT_SYS W_MOT_CMDS1/MOTOR_sys/MOTOR_2 ==
  note: motor with PROPELLER
  w_CMD : Inport
  Bus Selector1 : BusSelector  OutputSignals=Elec.i,TQ_mot.Kt_i
  Lift : Scope  NumInputPorts=3
  MOTOR_PARAMS_STRUCT : Subsystem  mask(DC motor){K=P_mot.Ka, B=P_mot.b, J=P_mot.I, GearRatio=1, R=P_mot.R, L=P_mot.L, Kb=P_mot.Ke, ID=P_mot.ID}
      mask prompts: K "Torque constant (N.m/A)"; B "Viscous friction co-efficient (N.m.s)"; J "Rotor Inertia (kg.m^2)"; GearRatio "Gear ratio (w_motor/w_wheel)"; R "Armature resistance (ohms)"; L "Armature Inductance (Henry)"; Kb "Back Emf constant (V.sec/rad)"; ID "Motor_ID  (#1 to #4)"
      mask help: DC motor
      mask DialogControl Container4 Prompt: Mechanical
      mask DialogControl Container9 Prompt: Electrical
      mask DialogControl Container32 Prompt: ID
      mask Display: disp('DC motor')
  Mux : Mux  Inputs=2
  PI_CONT : pid_lib/PID Controller  Controller=PI  Form=Parallel  TimeDomain=Continuous-time  UseExternalTs=off  SampleTime=-1  IntegratorMethod=Forward Euler  FilterMethod=Forward Euler  ControllerParametersSource=internal  P=2.97678216835849  I=24.9655384194189  D=-0.0417302954853434  UseFilter=on  N=6.67624174583517  TunerSelectOption=Transfer Function Based (PID Tuner App)  InitialConditionSource=internal  InitialConditionForIntegrator=0  InitialConditionForFilter=0  DifferentiatorICPrevScaledInput=0  ExternalReset=none  TrackingMode=off  Kt=1  LimitOutput=off  SatLimitsSource=internal  UpperSaturationLimit=inf  LowerSaturationLimit=-inf  LinearizeAsGain=on  AntiWindupMode=none  Kb=1  POutMin=[]  POutMax=[]  IOutMin=[]  IOutMax=[]  DOutMin=[]  DOutMax=[]  NOutMin=[]  NOutMax=[]  SumOutMin=[]  SumOutMax=[]  SaturationOutMin=[]  SaturationOutMax=[]  PParamMin=[]  PParamMax=[]  IParamMin=[]  IParamMax=[]  DParamMin=[]  DParamMax=[]  NParamMin=[]  NParamMax=[]  KbParamMin=[]  KbParamMax=[]  KtParamMin=[]  KtParamMax=[]  KbOutMin=[]  KbOutMax=[]  KtOutMin=[]  KtOutMax=[]  IntegratorOutMin=[]  IntegratorOutMax=[]  FilterOutMin=[]  FilterOutMax=[]  SumI1OutMin=[]  SumI1OutMax=[]  SumI2OutMin=[]  SumI2OutMax=[]  SumI3OutMin=[]  SumI3OutMax=[]  SumI4OutMin=[]  SumI4OutMax=[]  SumDOutMin=[]  SumDOutMax=[]  DifferentiatorOutMin=[]  DifferentiatorOutMax=[]  FilterDiffOutCoefMin=[]  FilterDiffOutCoefMax=[]  ReciprocalOutMin=[]  ReciprocalOutMax=[]  SumDenOutMin=[]  SumDenOutMax=[]  SumNumOutMin=[]  SumNumOutMax=[]  DivideOutMin=[]  DivideOutMax=[]  UdiffTsProdOutMin=[]  UdiffTsProdOutMax=[]  NTsProdOutMin=[]  NTsProdOutMax=[]  UintegralTsProdOutMin=[]  UintegralTsProdOutMax=[]  UngainTsProdOutMin=[]  UngainTsProdOutMax=[]  IntegratorContinuousStateAttributes=''  IntegratorStateMustResolveToSignalObject=off  IntegratorRTWStateStorageClass=Auto  FilterContinuousStateAttributes=''  FilterStateMustResolveToSignalObject=off  FilterRTWStateStorageClass=Auto  ParallelPVariant=InternalParameters  IdealPVariant=Disabled  IVariant=InternalParameters  DVariant=Disabled  IntegratorVariant=Continuous  SatVariant=Disabled  AWVariant=Passthrough  PCopyVariant=Disabled  TRVariant=Disabled  FdbkBlocksVariant=Forward  IdealPFdbkVariant=Disabled  SatFdbkVariant=Disabled  DerivativeFilterVariant=Disabled  NVariant=Disabled  NCopyVariant=Disabled_SignalSpec  FilterICVariant=Disabled  IntegratorICVariant=InternalICs  ExternalResetVariant=Disabled  TRSumVariant=Passthrough  SumFdbkVariant=Disabled  SumVariant=Sum_PI  TsampFilterVariant=InternalTs  TsampNgainVariant=Passthrough  TsampIntegralVariant=Passthrough  ExternalSaturationOutDataTypeStr=Inherit: Same as second input
  RPS_Lift_TG_drag : Scope  NumInputPorts=3
  Scope3 : Scope  NumInputPorts=4
  Sum1 : Sum  Inputs=|+-
  Terminator : Terminator
  VOLTAGE Saturation : Saturate  UpperLimit=P_elec.V_mot_max  LowerLimit=P_elec.V_mot_min
      settings: AttributesFormatString=|
      | Vmax = %<UpperLimit>
      | Vmin = %<LowerLimit>
  prefilter : Subsystem  mask(Derivative Estimation){wn=2*pi*5, p=1}
      mask prompts: wn "Natural frequency, wn (rad/sec)"; p "Damping ratio, p"
      mask help:
      | A simple derivative estimator using a 2nd order representation between input and output.
      |
      | The integrators use a discrete FORWARd Euler rule, and a sample time needs to be specified.
      mask init:
      | str1 = sprintf('wn = %.2f', wn);
      | str2 = sprintf('p  = %.2f', p);
      | %str3 = sprintf('dt = %.2f', dt);
      | %str = char(str1,str2,str3);
      | %str3 = sprintf('dt = %.2f', dt);
      | str = char(str1,str2);
      mask Display: disp(str)
  w_to_RPS : Subsystem
      mask Display: fprintf('w(rad/sec)\nto\nRPS')
  w_to_RPS1 : Subsystem
      mask Display: fprintf('w(rad/sec)\nto\nRPS')
  w_to_TQ_drag : Subsystem  mask(w_to_TQdrag){k=P_one_prop.TWIST_per_w2}
      mask prompts: k "k (N/ ( rad/sec)^2 )"
      mask help:
      | Convert angular speed w(rad/sec) into drag TORQUE,  M (N.m).
      | A simple quadratic rule is used:
      |
      | M = k * w^2
  w_to_Thrust : Subsystem  mask(w_to_thrust){k=P_one_prop.LIFT_per_w2}
      mask prompts: k "k (N/ ( rad/sec)^2 )"
      mask help:
      | Convert angular speed w(rad/sec) into lift thrust F (N).
      | A simple quadratic rule is used:
      |
      | F = k * w^2
  w : Outport  VectorParamsAs1DForOutWhenUnconnected=off
  wires:
  VOLTAGE Saturation/1 -> Lift/1, MOTOR_PARAMS_STRUCT/1(V)  "VOLTS"
  [TQdrag] -> RPS_Lift_TG_drag/3  "TQdrag"
  Sum1/1 -> PI_CONT/1
  w_to_TQ_drag/1(M) -> [TQdrag], MOTOR_PARAMS_STRUCT/2(TQ_LOAD), Scope3/4
  [LIFT] -> RPS_Lift_TG_drag/2  "LIFT"
  [wRPS_YES_prop] -> RPS_Lift_TG_drag/1  "RPS"
  w_to_Thrust/1(F) -> [LIFT]
  w_to_RPS/1(RPS) -> [wRPS_YES_prop], Scope3/1  "RPS"
  Bus Selector1/1 -> Scope3/2  "<i>"
  MOTOR_PARAMS_STRUCT/2(mot_bus) -> Bus Selector1/1
  Bus Selector1/2 -> Scope3/3  "<Kt_i>"
  MOTOR_PARAMS_STRUCT/1(w_motor) -> w_to_RPS/1(w), [w], w/1, w_to_Thrust/1(w), w_to_TQ_drag/1(w)
  [w] -> Sum1/2
  [LIFT] -> Lift/2  "LIFT"
  Mux/1 -> w_to_RPS1/1(w)  "w"
  [w] -> Mux/2
  w_to_RPS1/1(RPS) -> Lift/3  "w_RPS"
  PI_CONT/1 -> VOLTAGE Saturation/1  "VOLTS"
  w_CMD/1 -> prefilter/1(U)  "w_rad_per_sec"
  prefilter/1(U_filt) -> Mux/1, Sum1/1
  prefilter/2(U_DOT) -> Terminator/1

== system bh_compare_hand_to_SM_quad_pend/CONT_SYS W_MOT_CMDS1/MOTOR_sys/MOTOR_3 ==
  note: motor with PROPELLER
  w_CMD : Inport
  Bus Selector1 : BusSelector  OutputSignals=Elec.i,TQ_mot.Kt_i
  Lift : Scope  NumInputPorts=3
  MOTOR_PARAMS_STRUCT : Subsystem  mask(DC motor){K=P_mot.Ka, B=P_mot.b, J=P_mot.I, GearRatio=1, R=P_mot.R, L=P_mot.L, Kb=P_mot.Ke, ID=P_mot.ID}
      mask prompts: K "Torque constant (N.m/A)"; B "Viscous friction co-efficient (N.m.s)"; J "Rotor Inertia (kg.m^2)"; GearRatio "Gear ratio (w_motor/w_wheel)"; R "Armature resistance (ohms)"; L "Armature Inductance (Henry)"; Kb "Back Emf constant (V.sec/rad)"; ID "Motor_ID  (#1 to #4)"
      mask help: DC motor
      mask DialogControl Container4 Prompt: Mechanical
      mask DialogControl Container9 Prompt: Electrical
      mask DialogControl Container32 Prompt: ID
      mask Display: disp('DC motor')
  Mux : Mux  Inputs=2
  PI_CONT : pid_lib/PID Controller  Controller=PI  Form=Parallel  TimeDomain=Continuous-time  UseExternalTs=off  SampleTime=-1  IntegratorMethod=Forward Euler  FilterMethod=Forward Euler  ControllerParametersSource=internal  P=2.97678216835849  I=24.9655384194189  D=-0.0417302954853434  UseFilter=on  N=6.67624174583517  TunerSelectOption=Transfer Function Based (PID Tuner App)  InitialConditionSource=internal  InitialConditionForIntegrator=0  InitialConditionForFilter=0  DifferentiatorICPrevScaledInput=0  ExternalReset=none  TrackingMode=off  Kt=1  LimitOutput=off  SatLimitsSource=internal  UpperSaturationLimit=inf  LowerSaturationLimit=-inf  LinearizeAsGain=on  AntiWindupMode=none  Kb=1  POutMin=[]  POutMax=[]  IOutMin=[]  IOutMax=[]  DOutMin=[]  DOutMax=[]  NOutMin=[]  NOutMax=[]  SumOutMin=[]  SumOutMax=[]  SaturationOutMin=[]  SaturationOutMax=[]  PParamMin=[]  PParamMax=[]  IParamMin=[]  IParamMax=[]  DParamMin=[]  DParamMax=[]  NParamMin=[]  NParamMax=[]  KbParamMin=[]  KbParamMax=[]  KtParamMin=[]  KtParamMax=[]  KbOutMin=[]  KbOutMax=[]  KtOutMin=[]  KtOutMax=[]  IntegratorOutMin=[]  IntegratorOutMax=[]  FilterOutMin=[]  FilterOutMax=[]  SumI1OutMin=[]  SumI1OutMax=[]  SumI2OutMin=[]  SumI2OutMax=[]  SumI3OutMin=[]  SumI3OutMax=[]  SumI4OutMin=[]  SumI4OutMax=[]  SumDOutMin=[]  SumDOutMax=[]  DifferentiatorOutMin=[]  DifferentiatorOutMax=[]  FilterDiffOutCoefMin=[]  FilterDiffOutCoefMax=[]  ReciprocalOutMin=[]  ReciprocalOutMax=[]  SumDenOutMin=[]  SumDenOutMax=[]  SumNumOutMin=[]  SumNumOutMax=[]  DivideOutMin=[]  DivideOutMax=[]  UdiffTsProdOutMin=[]  UdiffTsProdOutMax=[]  NTsProdOutMin=[]  NTsProdOutMax=[]  UintegralTsProdOutMin=[]  UintegralTsProdOutMax=[]  UngainTsProdOutMin=[]  UngainTsProdOutMax=[]  IntegratorContinuousStateAttributes=''  IntegratorStateMustResolveToSignalObject=off  IntegratorRTWStateStorageClass=Auto  FilterContinuousStateAttributes=''  FilterStateMustResolveToSignalObject=off  FilterRTWStateStorageClass=Auto  ParallelPVariant=InternalParameters  IdealPVariant=Disabled  IVariant=InternalParameters  DVariant=Disabled  IntegratorVariant=Continuous  SatVariant=Disabled  AWVariant=Passthrough  PCopyVariant=Disabled  TRVariant=Disabled  FdbkBlocksVariant=Forward  IdealPFdbkVariant=Disabled  SatFdbkVariant=Disabled  DerivativeFilterVariant=Disabled  NVariant=Disabled  NCopyVariant=Disabled_SignalSpec  FilterICVariant=Disabled  IntegratorICVariant=InternalICs  ExternalResetVariant=Disabled  TRSumVariant=Passthrough  SumFdbkVariant=Disabled  SumVariant=Sum_PI  TsampFilterVariant=InternalTs  TsampNgainVariant=Passthrough  TsampIntegralVariant=Passthrough  ExternalSaturationOutDataTypeStr=Inherit: Same as second input
  RPS_Lift_TG_drag : Scope  NumInputPorts=3
  Scope3 : Scope  NumInputPorts=4
  Sum1 : Sum  Inputs=|+-
  Terminator : Terminator
  VOLTAGE Saturation : Saturate  UpperLimit=P_elec.V_mot_max  LowerLimit=P_elec.V_mot_min
      settings: AttributesFormatString=|
      | Vmax = %<UpperLimit>
      | Vmin = %<LowerLimit>
  prefilter : Subsystem  mask(Derivative Estimation){wn=2*pi*5, p=1}
      mask prompts: wn "Natural frequency, wn (rad/sec)"; p "Damping ratio, p"
      mask help:
      | A simple derivative estimator using a 2nd order representation between input and output.
      |
      | The integrators use a discrete FORWARd Euler rule, and a sample time needs to be specified.
      mask init:
      | str1 = sprintf('wn = %.2f', wn);
      | str2 = sprintf('p  = %.2f', p);
      | %str3 = sprintf('dt = %.2f', dt);
      | %str = char(str1,str2,str3);
      | %str3 = sprintf('dt = %.2f', dt);
      | str = char(str1,str2);
      mask Display: disp(str)
  w_to_RPS : Subsystem
      mask Display: fprintf('w(rad/sec)\nto\nRPS')
  w_to_RPS1 : Subsystem
      mask Display: fprintf('w(rad/sec)\nto\nRPS')
  w_to_TQ_drag : Subsystem  mask(w_to_TQdrag){k=P_one_prop.TWIST_per_w2}
      mask prompts: k "k (N/ ( rad/sec)^2 )"
      mask help:
      | Convert angular speed w(rad/sec) into drag TORQUE,  M (N.m).
      | A simple quadratic rule is used:
      |
      | M = k * w^2
  w_to_Thrust : Subsystem  mask(w_to_thrust){k=P_one_prop.LIFT_per_w2}
      mask prompts: k "k (N/ ( rad/sec)^2 )"
      mask help:
      | Convert angular speed w(rad/sec) into lift thrust F (N).
      | A simple quadratic rule is used:
      |
      | F = k * w^2
  w : Outport  VectorParamsAs1DForOutWhenUnconnected=off
  wires:
  VOLTAGE Saturation/1 -> Lift/1, MOTOR_PARAMS_STRUCT/1(V)  "VOLTS"
  [TQdrag] -> RPS_Lift_TG_drag/3  "TQdrag"
  Sum1/1 -> PI_CONT/1
  w_to_TQ_drag/1(M) -> [TQdrag], MOTOR_PARAMS_STRUCT/2(TQ_LOAD), Scope3/4
  [LIFT] -> RPS_Lift_TG_drag/2  "LIFT"
  [wRPS_YES_prop] -> RPS_Lift_TG_drag/1  "RPS"
  w_to_Thrust/1(F) -> [LIFT]
  w_to_RPS/1(RPS) -> [wRPS_YES_prop], Scope3/1  "RPS"
  Bus Selector1/1 -> Scope3/2  "<i>"
  MOTOR_PARAMS_STRUCT/2(mot_bus) -> Bus Selector1/1
  Bus Selector1/2 -> Scope3/3  "<Kt_i>"
  MOTOR_PARAMS_STRUCT/1(w_motor) -> w_to_RPS/1(w), [w], w/1, w_to_Thrust/1(w), w_to_TQ_drag/1(w)
  [w] -> Sum1/2
  [LIFT] -> Lift/2  "LIFT"
  Mux/1 -> w_to_RPS1/1(w)  "w"
  [w] -> Mux/2
  w_to_RPS1/1(RPS) -> Lift/3  "w_RPS"
  PI_CONT/1 -> VOLTAGE Saturation/1  "VOLTS"
  w_CMD/1 -> prefilter/1(U)  "w_rad_per_sec"
  prefilter/1(U_filt) -> Mux/1, Sum1/1
  prefilter/2(U_DOT) -> Terminator/1

== system bh_compare_hand_to_SM_quad_pend/CONT_SYS W_MOT_CMDS1/MOTOR_sys/MOTOR_4 ==
  note: motor with PROPELLER
  w_CMD : Inport
  Bus Selector1 : BusSelector  OutputSignals=Elec.i,TQ_mot.Kt_i
  Lift : Scope  NumInputPorts=3
  MOTOR_PARAMS_STRUCT : Subsystem  mask(DC motor){K=P_mot.Ka, B=P_mot.b, J=P_mot.I, GearRatio=1, R=P_mot.R, L=P_mot.L, Kb=P_mot.Ke, ID=P_mot.ID}
      mask prompts: K "Torque constant (N.m/A)"; B "Viscous friction co-efficient (N.m.s)"; J "Rotor Inertia (kg.m^2)"; GearRatio "Gear ratio (w_motor/w_wheel)"; R "Armature resistance (ohms)"; L "Armature Inductance (Henry)"; Kb "Back Emf constant (V.sec/rad)"; ID "Motor_ID  (#1 to #4)"
      mask help: DC motor
      mask DialogControl Container4 Prompt: Mechanical
      mask DialogControl Container9 Prompt: Electrical
      mask DialogControl Container32 Prompt: ID
      mask Display: disp('DC motor')
  Mux : Mux  Inputs=2
  PI_CONT : pid_lib/PID Controller  Controller=PI  Form=Parallel  TimeDomain=Continuous-time  UseExternalTs=off  SampleTime=-1  IntegratorMethod=Forward Euler  FilterMethod=Forward Euler  ControllerParametersSource=internal  P=2.97678216835849  I=24.9655384194189  D=-0.0417302954853434  UseFilter=on  N=6.67624174583517  TunerSelectOption=Transfer Function Based (PID Tuner App)  InitialConditionSource=internal  InitialConditionForIntegrator=0  InitialConditionForFilter=0  DifferentiatorICPrevScaledInput=0  ExternalReset=none  TrackingMode=off  Kt=1  LimitOutput=off  SatLimitsSource=internal  UpperSaturationLimit=inf  LowerSaturationLimit=-inf  LinearizeAsGain=on  AntiWindupMode=none  Kb=1  POutMin=[]  POutMax=[]  IOutMin=[]  IOutMax=[]  DOutMin=[]  DOutMax=[]  NOutMin=[]  NOutMax=[]  SumOutMin=[]  SumOutMax=[]  SaturationOutMin=[]  SaturationOutMax=[]  PParamMin=[]  PParamMax=[]  IParamMin=[]  IParamMax=[]  DParamMin=[]  DParamMax=[]  NParamMin=[]  NParamMax=[]  KbParamMin=[]  KbParamMax=[]  KtParamMin=[]  KtParamMax=[]  KbOutMin=[]  KbOutMax=[]  KtOutMin=[]  KtOutMax=[]  IntegratorOutMin=[]  IntegratorOutMax=[]  FilterOutMin=[]  FilterOutMax=[]  SumI1OutMin=[]  SumI1OutMax=[]  SumI2OutMin=[]  SumI2OutMax=[]  SumI3OutMin=[]  SumI3OutMax=[]  SumI4OutMin=[]  SumI4OutMax=[]  SumDOutMin=[]  SumDOutMax=[]  DifferentiatorOutMin=[]  DifferentiatorOutMax=[]  FilterDiffOutCoefMin=[]  FilterDiffOutCoefMax=[]  ReciprocalOutMin=[]  ReciprocalOutMax=[]  SumDenOutMin=[]  SumDenOutMax=[]  SumNumOutMin=[]  SumNumOutMax=[]  DivideOutMin=[]  DivideOutMax=[]  UdiffTsProdOutMin=[]  UdiffTsProdOutMax=[]  NTsProdOutMin=[]  NTsProdOutMax=[]  UintegralTsProdOutMin=[]  UintegralTsProdOutMax=[]  UngainTsProdOutMin=[]  UngainTsProdOutMax=[]  IntegratorContinuousStateAttributes=''  IntegratorStateMustResolveToSignalObject=off  IntegratorRTWStateStorageClass=Auto  FilterContinuousStateAttributes=''  FilterStateMustResolveToSignalObject=off  FilterRTWStateStorageClass=Auto  ParallelPVariant=InternalParameters  IdealPVariant=Disabled  IVariant=InternalParameters  DVariant=Disabled  IntegratorVariant=Continuous  SatVariant=Disabled  AWVariant=Passthrough  PCopyVariant=Disabled  TRVariant=Disabled  FdbkBlocksVariant=Forward  IdealPFdbkVariant=Disabled  SatFdbkVariant=Disabled  DerivativeFilterVariant=Disabled  NVariant=Disabled  NCopyVariant=Disabled_SignalSpec  FilterICVariant=Disabled  IntegratorICVariant=InternalICs  ExternalResetVariant=Disabled  TRSumVariant=Passthrough  SumFdbkVariant=Disabled  SumVariant=Sum_PI  TsampFilterVariant=InternalTs  TsampNgainVariant=Passthrough  TsampIntegralVariant=Passthrough  ExternalSaturationOutDataTypeStr=Inherit: Same as second input
  RPS_Lift_TG_drag : Scope  NumInputPorts=3
  Scope3 : Scope  NumInputPorts=4
  Sum1 : Sum  Inputs=|+-
  Terminator : Terminator
  VOLTAGE Saturation : Saturate  UpperLimit=P_elec.V_mot_max  LowerLimit=P_elec.V_mot_min
      settings: AttributesFormatString=|
      | Vmax = %<UpperLimit>
      | Vmin = %<LowerLimit>
  prefilter : Subsystem  mask(Derivative Estimation){wn=2*pi*5, p=1}
      mask prompts: wn "Natural frequency, wn (rad/sec)"; p "Damping ratio, p"
      mask help:
      | A simple derivative estimator using a 2nd order representation between input and output.
      |
      | The integrators use a discrete FORWARd Euler rule, and a sample time needs to be specified.
      mask init:
      | str1 = sprintf('wn = %.2f', wn);
      | str2 = sprintf('p  = %.2f', p);
      | %str3 = sprintf('dt = %.2f', dt);
      | %str = char(str1,str2,str3);
      | %str3 = sprintf('dt = %.2f', dt);
      | str = char(str1,str2);
      mask Display: disp(str)
  w_to_RPS : Subsystem
      mask Display: fprintf('w(rad/sec)\nto\nRPS')
  w_to_RPS1 : Subsystem
      mask Display: fprintf('w(rad/sec)\nto\nRPS')
  w_to_TQ_drag : Subsystem  mask(w_to_TQdrag){k=P_one_prop.TWIST_per_w2}
      mask prompts: k "k (N/ ( rad/sec)^2 )"
      mask help:
      | Convert angular speed w(rad/sec) into drag TORQUE,  M (N.m).
      | A simple quadratic rule is used:
      |
      | M = k * w^2
  w_to_Thrust : Subsystem  mask(w_to_thrust){k=P_one_prop.LIFT_per_w2}
      mask prompts: k "k (N/ ( rad/sec)^2 )"
      mask help:
      | Convert angular speed w(rad/sec) into lift thrust F (N).
      | A simple quadratic rule is used:
      |
      | F = k * w^2
  w : Outport  VectorParamsAs1DForOutWhenUnconnected=off
  wires:
  VOLTAGE Saturation/1 -> Lift/1, MOTOR_PARAMS_STRUCT/1(V)  "VOLTS"
  [TQdrag] -> RPS_Lift_TG_drag/3  "TQdrag"
  Sum1/1 -> PI_CONT/1
  w_to_TQ_drag/1(M) -> [TQdrag], MOTOR_PARAMS_STRUCT/2(TQ_LOAD), Scope3/4
  [LIFT] -> RPS_Lift_TG_drag/2  "LIFT"
  [wRPS_YES_prop] -> RPS_Lift_TG_drag/1  "RPS"
  w_to_Thrust/1(F) -> [LIFT]
  w_to_RPS/1(RPS) -> [wRPS_YES_prop], Scope3/1  "RPS"
  Bus Selector1/1 -> Scope3/2  "<i>"
  MOTOR_PARAMS_STRUCT/2(mot_bus) -> Bus Selector1/1
  Bus Selector1/2 -> Scope3/3  "<Kt_i>"
  MOTOR_PARAMS_STRUCT/1(w_motor) -> w_to_RPS/1(w), [w], w/1, w_to_Thrust/1(w), w_to_TQ_drag/1(w)
  [w] -> Sum1/2
  [LIFT] -> Lift/2  "LIFT"
  Mux/1 -> w_to_RPS1/1(w)  "w"
  [w] -> Mux/2
  w_to_RPS1/1(RPS) -> Lift/3  "w_RPS"
  PI_CONT/1 -> VOLTAGE Saturation/1  "VOLTS"
  w_CMD/1 -> prefilter/1(U)  "w_rad_per_sec"
  prefilter/1(U_filt) -> Mux/1, Sum1/1
  prefilter/2(U_DOT) -> Terminator/1

== system bh_compare_hand_to_SM_quad_pend/CONT_SYS W_MOT_CMDS1/MOTOR_sys/w_MUX ==
  W_CMD : Inport
  W : Inport  Port=2
  Demux1 : Demux
  Demux2 : Demux
  Mux{,1..3} (4 alike) : Mux  Inputs=2
  w1 : Outport  VectorParamsAs1DForOutWhenUnconnected=off
  w2 : Outport  Port=2  VectorParamsAs1DForOutWhenUnconnected=off
  w3 : Outport  Port=3  VectorParamsAs1DForOutWhenUnconnected=off
  w4 : Outport  Port=4  VectorParamsAs1DForOutWhenUnconnected=off
  wires:
  W_CMD/1 -> Demux2/1
  W/1 -> Demux1/1
  Mux/1 -> w1/1
  Mux1/1 -> w2/1
  Mux3/1 -> w4/1
  Mux2/1 -> w3/1
  Demux2/1 -> Mux/1
  Demux2/2 -> Mux1/1
  Demux2/3 -> Mux2/1
  Demux2/4 -> Mux3/1
  Demux1/1 -> Mux/2
  Demux1/2 -> Mux1/2
  Demux1/3 -> Mux2/2
  Demux1/4 -> Mux3/2

== system bh_compare_hand_to_SM_quad_pend/CONT_SYS W_MOT_CMDS2/PRE_FILTERS/prefilter ==
  note: Y = U *     wn^2/( s^2 + 2*p*wn*s + wn^2)
      | Y*( s^2 + 2*p*wn*s + wn^2) = U * wn^2
      |
      | y'' + y'*2*p*wn + y*wn^2 = U*wn^2
  U : Inport
  Gain : Gain  Gain=2*p*wn
  Gain1 : Gain  Gain=wn^2
  Gain2 : Gain  Gain=wn^2
  Integrator : Integrator
  Integrator1 : Integrator
  Sum : Sum  Inputs=|+--
  U_filt : Outport  VectorParamsAs1DForOutWhenUnconnected=off
  U_DOT : Outport  Port=2  VectorParamsAs1DForOutWhenUnconnected=off
  wires:
  Integrator/1 -> Integrator1/1, [Y_DOT], Gain/1  "y_dot"
  Sum/1 -> Integrator/1  "y_dot_dot"
  Integrator1/1 -> Gain1/1, U_filt/1  "y"
  U/1 -> Gain2/1
  Gain2/1 -> Sum/1
  Gain/1 -> Sum/3
  Gain1/1 -> Sum/2
  [Y_DOT] -> U_DOT/1

== system bh_compare_hand_to_SM_quad_pend/CONT_SYS W_MOT_CMDS2/PRE_FILTERS/prefilter1 ==
  note: Y = U *     wn^2/( s^2 + 2*p*wn*s + wn^2)
      | Y*( s^2 + 2*p*wn*s + wn^2) = U * wn^2
      |
      | y'' + y'*2*p*wn + y*wn^2 = U*wn^2
  U : Inport
  Gain : Gain  Gain=2*p*wn
  Gain1 : Gain  Gain=wn^2
  Gain2 : Gain  Gain=wn^2
  Integrator : Integrator
  Integrator1 : Integrator
  Sum : Sum  Inputs=|+--
  U_filt : Outport  VectorParamsAs1DForOutWhenUnconnected=off
  U_DOT : Outport  Port=2  VectorParamsAs1DForOutWhenUnconnected=off
  wires:
  Integrator/1 -> Integrator1/1, [Y_DOT], Gain/1  "y_dot"
  Sum/1 -> Integrator/1  "y_dot_dot"
  Integrator1/1 -> Gain1/1, U_filt/1  "y"
  U/1 -> Gain2/1
  Gain2/1 -> Sum/1
  Gain/1 -> Sum/3
  Gain1/1 -> Sum/2
  [Y_DOT] -> U_DOT/1

== system bh_compare_hand_to_SM_quad_pend/CONT_SYS W_MOT_CMDS2/PRE_FILTERS/prefilter2 ==
  note: Y = U *     wn^2/( s^2 + 2*p*wn*s + wn^2)
      | Y*( s^2 + 2*p*wn*s + wn^2) = U * wn^2
      |
      | y'' + y'*2*p*wn + y*wn^2 = U*wn^2
  U : Inport
  Gain : Gain  Gain=2*p*wn
  Gain1 : Gain  Gain=wn^2
  Gain2 : Gain  Gain=wn^2
  Integrator : Integrator
  Integrator1 : Integrator
  Sum : Sum  Inputs=|+--
  U_filt : Outport  VectorParamsAs1DForOutWhenUnconnected=off
  U_DOT : Outport  Port=2  VectorParamsAs1DForOutWhenUnconnected=off
  wires:
  Integrator/1 -> Integrator1/1, [Y_DOT], Gain/1  "y_dot"
  Sum/1 -> Integrator/1  "y_dot_dot"
  Integrator1/1 -> Gain1/1, U_filt/1  "y"
  U/1 -> Gain2/1
  Gain2/1 -> Sum/1
  Gain/1 -> Sum/3
  Gain1/1 -> Sum/2
  [Y_DOT] -> U_DOT/1
